simulink model "OORT"  (Simulink 7.6)
settings: Solver=ode3  SolverMode=SingleTasking  StartTime=0.0  StopTime=1.2  FixedStep=2e-5  RelTol=1e-4  AbsTol=1e-6
undefined symbols (not defined in the file or in its folder): DAB, den, elements, num
libraries: powerlib x179, powerlib_extras x6
(part 3 of 4)

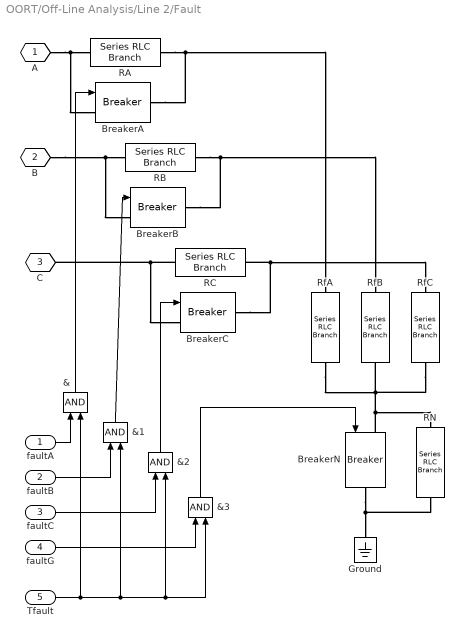
== system OORT/Off-Line Analysis/Line 2/Fault ==
  faultA : Inport
  faultB : Inport  Port=2
  faultC : Inport  Port=3
  faultG : Inport  Port=4
  Tfault : Inport  Port=5
  &{,1..3} (4 alike) : Logic
  BreakerA : powerlib/Elements/Breaker  DialogController=POWERSYS.PowerSysDialog  SystemSampleTime=-1  BreakerResistance=0.01  InitialState=0  SnubberResistance=1e6  SnubberCapacitance=inf  SwitchingTimes="[ 1/60  5/60 ]"  External=on  Measurements=None  MoreParameters=off  NoBreakLoop=off
  BreakerB : powerlib/Elements/Breaker  DialogController=POWERSYS.PowerSysDialog  SystemSampleTime=-1  BreakerResistance=0.01  InitialState=0  SnubberResistance=1e6  SnubberCapacitance=inf  SwitchingTimes="[ 1/60  5/60 ]"  External=on  Measurements=None  MoreParameters=off  NoBreakLoop=off
  BreakerC : powerlib/Elements/Breaker  DialogController=POWERSYS.PowerSysDialog  SystemSampleTime=-1  BreakerResistance=0.01  InitialState=0  SnubberResistance=1e6  SnubberCapacitance=inf  SwitchingTimes="[ 1/60  5/60 ]"  External=on  Measurements=None  MoreParameters=off  NoBreakLoop=off
  BreakerN : powerlib/Elements/Breaker  DialogController=POWERSYS.PowerSysDialog  SystemSampleTime=-1  BreakerResistance=0.01  InitialState=0  SnubberResistance=1e6  SnubberCapacitance=inf  SwitchingTimes="[ 1/60  5/60 ]"  External=on  Measurements=None  MoreParameters=off  NoBreakLoop=off
  Ground : powerlib/Elements/Ground  DialogController=POWERSYS.PowerSysDialog  PhysicalDomain=powersysdomain  SubClassName=unknown  LeftPortType=p1  RightPortType=p1  LConnTagsString=a
  RA : powerlib/Elements/Series RLC Branch  DialogController=POWERSYS.PowerSysDialog  PhysicalDomain=powersysdomain  SubClassName=unknown  LeftPortType=p1  RightPortType=p1  LConnTagsString=__new0  RConnTagsString=__new0  BranchType=R  Resistance=10000  Inductance=1e-3  SetiL0=off  InitialCurrent=0  Capacitance=1e-6  Setx0=off  InitialVoltage=0  Measurements=None
  RB : powerlib/Elements/Series RLC Branch  DialogController=POWERSYS.PowerSysDialog  PhysicalDomain=powersysdomain  SubClassName=unknown  LeftPortType=p1  RightPortType=p1  LConnTagsString=__new0  RConnTagsString=__new0  BranchType=R  Resistance=10000  Inductance=1e-3  SetiL0=off  InitialCurrent=0  Capacitance=1e-6  Setx0=off  InitialVoltage=0  Measurements=None
  RC : powerlib/Elements/Series RLC Branch  DialogController=POWERSYS.PowerSysDialog  PhysicalDomain=powersysdomain  SubClassName=unknown  LeftPortType=p1  RightPortType=p1  LConnTagsString=__new0  RConnTagsString=__new0  BranchType=R  Resistance=10000  Inductance=1e-3  SetiL0=off  InitialCurrent=0  Capacitance=1e-6  Setx0=off  InitialVoltage=0  Measurements=None
  RN : powerlib/Elements/Series RLC Branch  DialogController=POWERSYS.PowerSysDialog  PhysicalDomain=powersysdomain  SubClassName=unknown  LeftPortType=p1  RightPortType=p1  LConnTagsString=__new0  RConnTagsString=__new0  BranchType=R  Resistance=10000  Inductance=1e-3  SetiL0=off  InitialCurrent=0  Capacitance=1e-6  Setx0=off  InitialVoltage=0  Measurements=None
  RfA : powerlib/Elements/Series RLC Branch  DialogController=POWERSYS.PowerSysDialog  PhysicalDomain=powersysdomain  SubClassName=unknown  LeftPortType=p1  RightPortType=p1  LConnTagsString=__new0  RConnTagsString=__new0  BranchType=R  Resistance=faultR  Inductance=1e-3  SetiL0=off  InitialCurrent=0  Capacitance=1e-6  Setx0=off  InitialVoltage=0  Measurements=None
  RfB : powerlib/Elements/Series RLC Branch  DialogController=POWERSYS.PowerSysDialog  PhysicalDomain=powersysdomain  SubClassName=unknown  LeftPortType=p1  RightPortType=p1  LConnTagsString=__new0  RConnTagsString=__new0  BranchType=R  Resistance=faultR  Inductance=1e-3  SetiL0=off  InitialCurrent=0  Capacitance=1e-6  Setx0=off  InitialVoltage=0  Measurements=None
  RfC : powerlib/Elements/Series RLC Branch  DialogController=POWERSYS.PowerSysDialog  PhysicalDomain=powersysdomain  SubClassName=unknown  LeftPortType=p1  RightPortType=p1  LConnTagsString=__new0  RConnTagsString=__new0  BranchType=R  Resistance=faultR  Inductance=1e-3  SetiL0=off  InitialCurrent=0  Capacitance=1e-6  Setx0=off  InitialVoltage=0  Measurements=None
  A : PMIOPort  Tag=PMCPort  Port=1  Side=Left
  B : PMIOPort  Tag=PMCPort  Port=2  Side=Left
  C : PMIOPort  Tag=PMCPort  Port=3  Side=Left
  wires:
  faultA/1 -> &/1
  faultB/1 -> &1/1
  faultC/1 -> &2/1
  faultG/1 -> &3/1
  Tfault/1 -> &3/2, &2/2, &1/2, &/2
  &3/1 -> BreakerN/1
  &/1 -> BreakerA/1
  &1/1 -> BreakerB/1
  &2/1 -> BreakerC/1
  connections:
  B/RConn1 -- RB/LConn1 -- BreakerB/LConn1
  A/RConn1 -- BreakerA/LConn1 -- RA/LConn1
  RC/LConn1 -- C/RConn1 -- BreakerC/LConn1
  BreakerC/RConn1 -- RC/RConn1 -- RfC/LConn1
  RB/RConn1 -- RfB/LConn1 -- BreakerB/RConn1
  RA/RConn1 -- RfA/LConn1 -- BreakerA/RConn1
  BreakerN/LConn1 -- RN/LConn1 -- RfB/RConn1 -- RfA/RConn1 -- RfC/RConn1
  BreakerN/RConn1 -- Ground/LConn1 -- RN/RConn1

== system OORT/Off-Line Analysis/Line 2/Fault Selector ==
  "  " : Constant  Value=faultType
  "  +" : Logic  Operator=OR  Inputs=7
  " +" : Logic  Operator=OR  Inputs=5
  + : Logic  Operator=OR  Inputs=5
  "+ " : Logic  Operator=OR  Inputs=6
  A-B-C : Fcn  Expr=(u(1)==8)
  A-B-C-G : Fcn  Expr=(u(1)==9)
  A-G : Fcn  Expr=(u(1)==1)
  B-C : Fcn  Expr=(u(1)==4)
  B-C-G : Fcn  Expr=(u(1)==5)
  B-G : Fcn  Expr=(u(1)==2)
  C-A : Fcn  Expr=(u(1)==6)
  C-A-G : Fcn  Expr=(u(1)==7)
  C-G : Fcn  Expr=(u(1)==3)
  faultA : Outport  InitialOutput=0
  faultB : Outport  Port=2  InitialOutput=0
  faultC : Outport  Port=3  InitialOutput=0
  faultG : Outport  Port=4  InitialOutput=0
  wires:
  "  "/1 -> C-G/1, A-G/1, B-G/1, B-C/1, C-A/1, C-A-G/1, A-B-C/1, A-B-C-G/1, B-C-G/1
  +/1 -> faultA/1
  " +"/1 -> faultB/1
  "  +"/1 -> faultC/1
  "+ "/1 -> faultG/1
  A-G/1 -> "+ "/1, +/1
  C-A/1 -> "  +"/4, +/2
  B-G/1 -> " +"/1, "+ "/2
  B-C/1 -> "  +"/2, " +"/2
  B-C-G/1 -> "  +"/3, "+ "/4, " +"/3
  C-G/1 -> "  +"/1, "+ "/3
  C-A-G/1 -> "  +"/5, "+ "/5, +/3
  A-B-C-G/1 -> " +"/5, "  +"/7, "+ "/6, +/5
  A-B-C/1 -> " +"/4, "  +"/6, +/4

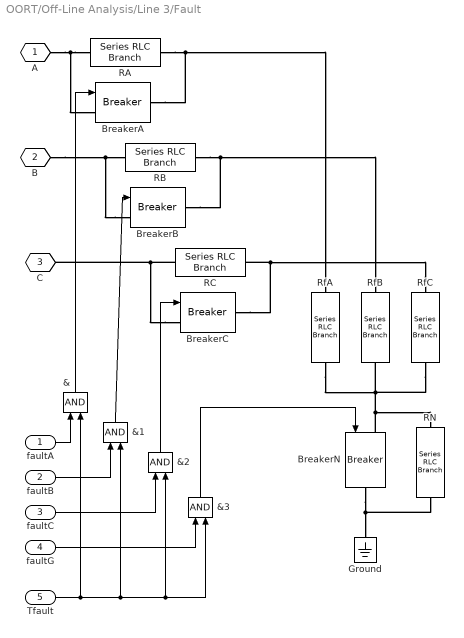
== system OORT/Off-Line Analysis/Line 3/Fault ==
  faultA : Inport
  faultB : Inport  Port=2
  faultC : Inport  Port=3
  faultG : Inport  Port=4
  Tfault : Inport  Port=5
  &{,1..3} (4 alike) : Logic
  BreakerA : powerlib/Elements/Breaker  DialogController=POWERSYS.PowerSysDialog  SystemSampleTime=-1  BreakerResistance=0.01  InitialState=0  SnubberResistance=1e6  SnubberCapacitance=inf  SwitchingTimes="[ 1/60  5/60 ]"  External=on  Measurements=None  MoreParameters=off  NoBreakLoop=off
  BreakerB : powerlib/Elements/Breaker  DialogController=POWERSYS.PowerSysDialog  SystemSampleTime=-1  BreakerResistance=0.01  InitialState=0  SnubberResistance=1e6  SnubberCapacitance=inf  SwitchingTimes="[ 1/60  5/60 ]"  External=on  Measurements=None  MoreParameters=off  NoBreakLoop=off
  BreakerC : powerlib/Elements/Breaker  DialogController=POWERSYS.PowerSysDialog  SystemSampleTime=-1  BreakerResistance=0.01  InitialState=0  SnubberResistance=1e6  SnubberCapacitance=inf  SwitchingTimes="[ 1/60  5/60 ]"  External=on  Measurements=None  MoreParameters=off  NoBreakLoop=off
  BreakerN : powerlib/Elements/Breaker  DialogController=POWERSYS.PowerSysDialog  SystemSampleTime=-1  BreakerResistance=0.01  InitialState=0  SnubberResistance=1e6  SnubberCapacitance=inf  SwitchingTimes="[ 1/60  5/60 ]"  External=on  Measurements=None  MoreParameters=off  NoBreakLoop=off
  Ground : powerlib/Elements/Ground  DialogController=POWERSYS.PowerSysDialog  PhysicalDomain=powersysdomain  SubClassName=unknown  LeftPortType=p1  RightPortType=p1  LConnTagsString=a
  RA : powerlib/Elements/Series RLC Branch  DialogController=POWERSYS.PowerSysDialog  PhysicalDomain=powersysdomain  SubClassName=unknown  LeftPortType=p1  RightPortType=p1  LConnTagsString=__new0  RConnTagsString=__new0  BranchType=R  Resistance=10000  Inductance=1e-3  SetiL0=off  InitialCurrent=0  Capacitance=1e-6  Setx0=off  InitialVoltage=0  Measurements=None
  RB : powerlib/Elements/Series RLC Branch  DialogController=POWERSYS.PowerSysDialog  PhysicalDomain=powersysdomain  SubClassName=unknown  LeftPortType=p1  RightPortType=p1  LConnTagsString=__new0  RConnTagsString=__new0  BranchType=R  Resistance=10000  Inductance=1e-3  SetiL0=off  InitialCurrent=0  Capacitance=1e-6  Setx0=off  InitialVoltage=0  Measurements=None
  RC : powerlib/Elements/Series RLC Branch  DialogController=POWERSYS.PowerSysDialog  PhysicalDomain=powersysdomain  SubClassName=unknown  LeftPortType=p1  RightPortType=p1  LConnTagsString=__new0  RConnTagsString=__new0  BranchType=R  Resistance=10000  Inductance=1e-3  SetiL0=off  InitialCurrent=0  Capacitance=1e-6  Setx0=off  InitialVoltage=0  Measurements=None
  RN : powerlib/Elements/Series RLC Branch  DialogController=POWERSYS.PowerSysDialog  PhysicalDomain=powersysdomain  SubClassName=unknown  LeftPortType=p1  RightPortType=p1  LConnTagsString=__new0  RConnTagsString=__new0  BranchType=R  Resistance=10000  Inductance=1e-3  SetiL0=off  InitialCurrent=0  Capacitance=1e-6  Setx0=off  InitialVoltage=0  Measurements=None
  RfA : powerlib/Elements/Series RLC Branch  DialogController=POWERSYS.PowerSysDialog  PhysicalDomain=powersysdomain  SubClassName=unknown  LeftPortType=p1  RightPortType=p1  LConnTagsString=__new0  RConnTagsString=__new0  BranchType=R  Resistance=faultR  Inductance=1e-3  SetiL0=off  InitialCurrent=0  Capacitance=1e-6  Setx0=off  InitialVoltage=0  Measurements=None
  RfB : powerlib/Elements/Series RLC Branch  DialogController=POWERSYS.PowerSysDialog  PhysicalDomain=powersysdomain  SubClassName=unknown  LeftPortType=p1  RightPortType=p1  LConnTagsString=__new0  RConnTagsString=__new0  BranchType=R  Resistance=faultR  Inductance=1e-3  SetiL0=off  InitialCurrent=0  Capacitance=1e-6  Setx0=off  InitialVoltage=0  Measurements=None
  RfC : powerlib/Elements/Series RLC Branch  DialogController=POWERSYS.PowerSysDialog  PhysicalDomain=powersysdomain  SubClassName=unknown  LeftPortType=p1  RightPortType=p1  LConnTagsString=__new0  RConnTagsString=__new0  BranchType=R  Resistance=faultR  Inductance=1e-3  SetiL0=off  InitialCurrent=0  Capacitance=1e-6  Setx0=off  InitialVoltage=0  Measurements=None
  A : PMIOPort  Tag=PMCPort  Port=1  Side=Left
  B : PMIOPort  Tag=PMCPort  Port=2  Side=Left
  C : PMIOPort  Tag=PMCPort  Port=3  Side=Left
  wires:
  &2/1 -> BreakerC/1
  &1/1 -> BreakerB/1
  &/1 -> BreakerA/1
  &3/1 -> BreakerN/1
  Tfault/1 -> &/2, &1/2, &2/2, &3/2
  faultG/1 -> &3/1
  faultC/1 -> &2/1
  faultB/1 -> &1/1
  faultA/1 -> &/1
  connections:
  RN/RConn1 -- Ground/LConn1 -- BreakerN/RConn1
  RfC/RConn1 -- RfA/RConn1 -- RfB/RConn1 -- RN/LConn1 -- BreakerN/LConn1
  BreakerA/RConn1 -- RfA/LConn1 -- RA/RConn1
  BreakerB/RConn1 -- RfB/LConn1 -- RB/RConn1
  RfC/LConn1 -- RC/RConn1 -- BreakerC/RConn1
  BreakerC/LConn1 -- C/RConn1 -- RC/LConn1
  RA/LConn1 -- BreakerA/LConn1 -- A/RConn1
  BreakerB/LConn1 -- RB/LConn1 -- B/RConn1

== system OORT/Off-Line Analysis/Line 3/Fault Selector ==
  "  " : Constant  Value=faultType
  "  +" : Logic  Operator=OR  Inputs=7
  " +" : Logic  Operator=OR  Inputs=5
  + : Logic  Operator=OR  Inputs=5
  "+ " : Logic  Operator=OR  Inputs=6
  A-B-C : Fcn  Expr=(u(1)==8)
  A-B-C-G : Fcn  Expr=(u(1)==9)
  A-G : Fcn  Expr=(u(1)==1)
  B-C : Fcn  Expr=(u(1)==4)
  B-C-G : Fcn  Expr=(u(1)==5)
  B-G : Fcn  Expr=(u(1)==2)
  C-A : Fcn  Expr=(u(1)==6)
  C-A-G : Fcn  Expr=(u(1)==7)
  C-G : Fcn  Expr=(u(1)==3)
  faultA : Outport  InitialOutput=0
  faultB : Outport  Port=2  InitialOutput=0
  faultC : Outport  Port=3  InitialOutput=0
  faultG : Outport  Port=4  InitialOutput=0
  wires:
  A-B-C/1 -> +/4, "  +"/6, " +"/4
  A-B-C-G/1 -> +/5, "+ "/6, "  +"/7, " +"/5
  C-A-G/1 -> +/3, "+ "/5, "  +"/5
  C-G/1 -> "+ "/3, "  +"/1
  B-C-G/1 -> " +"/3, "+ "/4, "  +"/3
  B-C/1 -> " +"/2, "  +"/2
  B-G/1 -> "+ "/2, " +"/1
  C-A/1 -> +/2, "  +"/4
  A-G/1 -> +/1, "+ "/1
  "+ "/1 -> faultG/1
  "  +"/1 -> faultC/1
  " +"/1 -> faultB/1
  +/1 -> faultA/1
  "  "/1 -> B-C-G/1, A-B-C-G/1, A-B-C/1, C-A-G/1, C-A/1, B-C/1, B-G/1, A-G/1, C-G/1

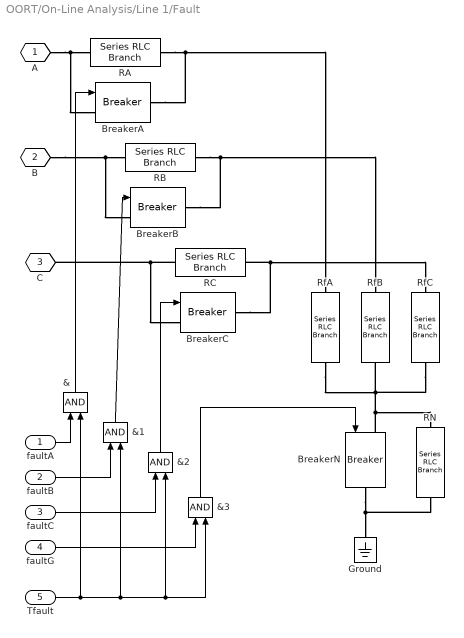
== system OORT/On-Line Analysis/Line 1/Fault ==
  faultA : Inport
  faultB : Inport  Port=2
  faultC : Inport  Port=3
  faultG : Inport  Port=4
  Tfault : Inport  Port=5
  &{,1..3} (4 alike) : Logic
  BreakerA : powerlib/Elements/Breaker  DialogController=POWERSYS.PowerSysDialog  SystemSampleTime=-1  BreakerResistance=0.01  InitialState=0  SnubberResistance=1e6  SnubberCapacitance=inf  SwitchingTimes="[ 1/60  5/60 ]"  External=on  Measurements=None  MoreParameters=off  NoBreakLoop=off
  BreakerB : powerlib/Elements/Breaker  DialogController=POWERSYS.PowerSysDialog  SystemSampleTime=-1  BreakerResistance=0.01  InitialState=0  SnubberResistance=1e6  SnubberCapacitance=inf  SwitchingTimes="[ 1/60  5/60 ]"  External=on  Measurements=None  MoreParameters=off  NoBreakLoop=off
  BreakerC : powerlib/Elements/Breaker  DialogController=POWERSYS.PowerSysDialog  SystemSampleTime=-1  BreakerResistance=0.01  InitialState=0  SnubberResistance=1e6  SnubberCapacitance=inf  SwitchingTimes="[ 1/60  5/60 ]"  External=on  Measurements=None  MoreParameters=off  NoBreakLoop=off
  BreakerN : powerlib/Elements/Breaker  DialogController=POWERSYS.PowerSysDialog  SystemSampleTime=-1  BreakerResistance=0.01  InitialState=0  SnubberResistance=1e6  SnubberCapacitance=inf  SwitchingTimes="[ 1/60  5/60 ]"  External=on  Measurements=None  MoreParameters=off  NoBreakLoop=off
  Ground : powerlib/Elements/Ground  DialogController=POWERSYS.PowerSysDialog  PhysicalDomain=powersysdomain  SubClassName=unknown  LeftPortType=p1  RightPortType=p1  LConnTagsString=a
  RA : powerlib/Elements/Series RLC Branch  DialogController=POWERSYS.PowerSysDialog  PhysicalDomain=powersysdomain  SubClassName=unknown  LeftPortType=p1  RightPortType=p1  LConnTagsString=__new0  RConnTagsString=__new0  BranchType=R  Resistance=10000  Inductance=1e-3  SetiL0=off  InitialCurrent=0  Capacitance=1e-6  Setx0=off  InitialVoltage=0  Measurements=None
  RB : powerlib/Elements/Series RLC Branch  DialogController=POWERSYS.PowerSysDialog  PhysicalDomain=powersysdomain  SubClassName=unknown  LeftPortType=p1  RightPortType=p1  LConnTagsString=__new0  RConnTagsString=__new0  BranchType=R  Resistance=10000  Inductance=1e-3  SetiL0=off  InitialCurrent=0  Capacitance=1e-6  Setx0=off  InitialVoltage=0  Measurements=None
  RC : powerlib/Elements/Series RLC Branch  DialogController=POWERSYS.PowerSysDialog  PhysicalDomain=powersysdomain  SubClassName=unknown  LeftPortType=p1  RightPortType=p1  LConnTagsString=__new0  RConnTagsString=__new0  BranchType=R  Resistance=10000  Inductance=1e-3  SetiL0=off  InitialCurrent=0  Capacitance=1e-6  Setx0=off  InitialVoltage=0  Measurements=None
  RN : powerlib/Elements/Series RLC Branch  DialogController=POWERSYS.PowerSysDialog  PhysicalDomain=powersysdomain  SubClassName=unknown  LeftPortType=p1  RightPortType=p1  LConnTagsString=__new0  RConnTagsString=__new0  BranchType=R  Resistance=10000  Inductance=1e-3  SetiL0=off  InitialCurrent=0  Capacitance=1e-6  Setx0=off  InitialVoltage=0  Measurements=None
  RfA : powerlib/Elements/Series RLC Branch  DialogController=POWERSYS.PowerSysDialog  PhysicalDomain=powersysdomain  SubClassName=unknown  LeftPortType=p1  RightPortType=p1  LConnTagsString=__new0  RConnTagsString=__new0  BranchType=R  Resistance=faultR  Inductance=1e-3  SetiL0=off  InitialCurrent=0  Capacitance=1e-6  Setx0=off  InitialVoltage=0  Measurements=None
  RfB : powerlib/Elements/Series RLC Branch  DialogController=POWERSYS.PowerSysDialog  PhysicalDomain=powersysdomain  SubClassName=unknown  LeftPortType=p1  RightPortType=p1  LConnTagsString=__new0  RConnTagsString=__new0  BranchType=R  Resistance=faultR  Inductance=1e-3  SetiL0=off  InitialCurrent=0  Capacitance=1e-6  Setx0=off  InitialVoltage=0  Measurements=None
  RfC : powerlib/Elements/Series RLC Branch  DialogController=POWERSYS.PowerSysDialog  PhysicalDomain=powersysdomain  SubClassName=unknown  LeftPortType=p1  RightPortType=p1  LConnTagsString=__new0  RConnTagsString=__new0  BranchType=R  Resistance=faultR  Inductance=1e-3  SetiL0=off  InitialCurrent=0  Capacitance=1e-6  Setx0=off  InitialVoltage=0  Measurements=None
  A : PMIOPort  Tag=PMCPort  Port=1  Side=Left
  B : PMIOPort  Tag=PMCPort  Port=2  Side=Left
  C : PMIOPort  Tag=PMCPort  Port=3  Side=Left
  wires:
  faultA/1 -> &/1
  faultB/1 -> &1/1
  faultC/1 -> &2/1
  faultG/1 -> &3/1
  Tfault/1 -> &3/2, &2/2, &1/2, &/2
  &3/1 -> BreakerN/1
  &/1 -> BreakerA/1
  &1/1 -> BreakerB/1
  &2/1 -> BreakerC/1
  connections:
  B/RConn1 -- RB/LConn1 -- BreakerB/LConn1
  A/RConn1 -- BreakerA/LConn1 -- RA/LConn1
  RC/LConn1 -- C/RConn1 -- BreakerC/LConn1
  BreakerC/RConn1 -- RC/RConn1 -- RfC/LConn1
  RB/RConn1 -- RfB/LConn1 -- BreakerB/RConn1
  RA/RConn1 -- RfA/LConn1 -- BreakerA/RConn1
  BreakerN/LConn1 -- RN/LConn1 -- RfB/RConn1 -- RfA/RConn1 -- RfC/RConn1
  BreakerN/RConn1 -- Ground/LConn1 -- RN/RConn1

== system OORT/On-Line Analysis/Line 1/Fault Selector ==
  "  " : Constant  Value=faultType
  "  +" : Logic  Operator=OR  Inputs=7
  " +" : Logic  Operator=OR  Inputs=5
  + : Logic  Operator=OR  Inputs=5
  "+ " : Logic  Operator=OR  Inputs=6
  A-B-C : Fcn  Expr=(u(1)==8)
  A-B-C-G : Fcn  Expr=(u(1)==9)
  A-G : Fcn  Expr=(u(1)==1)
  B-C : Fcn  Expr=(u(1)==4)
  B-C-G : Fcn  Expr=(u(1)==5)
  B-G : Fcn  Expr=(u(1)==2)
  C-A : Fcn  Expr=(u(1)==6)
  C-A-G : Fcn  Expr=(u(1)==7)
  C-G : Fcn  Expr=(u(1)==3)
  faultA : Outport  InitialOutput=0
  faultB : Outport  Port=2  InitialOutput=0
  faultC : Outport  Port=3  InitialOutput=0
  faultG : Outport  Port=4  InitialOutput=0
  wires:
  "  "/1 -> C-G/1, A-G/1, B-G/1, B-C/1, C-A/1, C-A-G/1, A-B-C/1, A-B-C-G/1, B-C-G/1
  +/1 -> faultA/1
  " +"/1 -> faultB/1
  "  +"/1 -> faultC/1
  "+ "/1 -> faultG/1
  A-G/1 -> "+ "/1, +/1
  C-A/1 -> "  +"/4, +/2
  B-G/1 -> " +"/1, "+ "/2
  B-C/1 -> "  +"/2, " +"/2
  B-C-G/1 -> "  +"/3, "+ "/4, " +"/3
  C-G/1 -> "  +"/1, "+ "/3
  C-A-G/1 -> "  +"/5, "+ "/5, +/3
  A-B-C-G/1 -> " +"/5, "  +"/7, "+ "/6, +/5
  A-B-C/1 -> " +"/4, "  +"/6, +/4

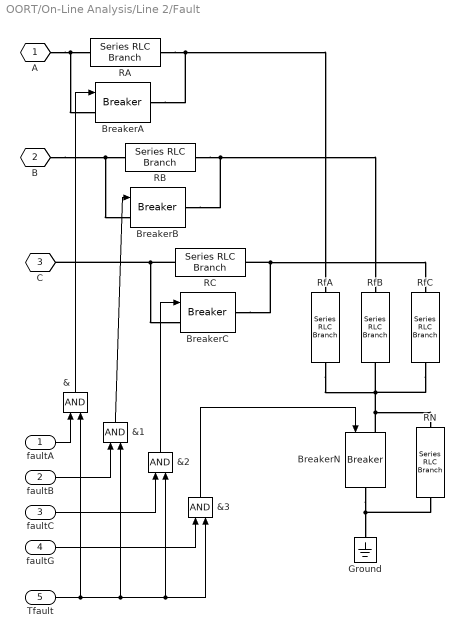
== system OORT/On-Line Analysis/Line 2/Fault ==
  faultA : Inport
  faultB : Inport  Port=2
  faultC : Inport  Port=3
  faultG : Inport  Port=4
  Tfault : Inport  Port=5
  &{,1..3} (4 alike) : Logic
  BreakerA : powerlib/Elements/Breaker  DialogController=POWERSYS.PowerSysDialog  SystemSampleTime=-1  BreakerResistance=0.01  InitialState=0  SnubberResistance=1e6  SnubberCapacitance=inf  SwitchingTimes="[ 1/60  5/60 ]"  External=on  Measurements=None  MoreParameters=off  NoBreakLoop=off
  BreakerB : powerlib/Elements/Breaker  DialogController=POWERSYS.PowerSysDialog  SystemSampleTime=-1  BreakerResistance=0.01  InitialState=0  SnubberResistance=1e6  SnubberCapacitance=inf  SwitchingTimes="[ 1/60  5/60 ]"  External=on  Measurements=None  MoreParameters=off  NoBreakLoop=off
  BreakerC : powerlib/Elements/Breaker  DialogController=POWERSYS.PowerSysDialog  SystemSampleTime=-1  BreakerResistance=0.01  InitialState=0  SnubberResistance=1e6  SnubberCapacitance=inf  SwitchingTimes="[ 1/60  5/60 ]"  External=on  Measurements=None  MoreParameters=off  NoBreakLoop=off
  BreakerN : powerlib/Elements/Breaker  DialogController=POWERSYS.PowerSysDialog  SystemSampleTime=-1  BreakerResistance=0.01  InitialState=0  SnubberResistance=1e6  SnubberCapacitance=inf  SwitchingTimes="[ 1/60  5/60 ]"  External=on  Measurements=None  MoreParameters=off  NoBreakLoop=off
  Ground : powerlib/Elements/Ground  DialogController=POWERSYS.PowerSysDialog  PhysicalDomain=powersysdomain  SubClassName=unknown  LeftPortType=p1  RightPortType=p1  LConnTagsString=a
  RA : powerlib/Elements/Series RLC Branch  DialogController=POWERSYS.PowerSysDialog  PhysicalDomain=powersysdomain  SubClassName=unknown  LeftPortType=p1  RightPortType=p1  LConnTagsString=__new0  RConnTagsString=__new0  BranchType=R  Resistance=10000  Inductance=1e-3  SetiL0=off  InitialCurrent=0  Capacitance=1e-6  Setx0=off  InitialVoltage=0  Measurements=None
  RB : powerlib/Elements/Series RLC Branch  DialogController=POWERSYS.PowerSysDialog  PhysicalDomain=powersysdomain  SubClassName=unknown  LeftPortType=p1  RightPortType=p1  LConnTagsString=__new0  RConnTagsString=__new0  BranchType=R  Resistance=10000  Inductance=1e-3  SetiL0=off  InitialCurrent=0  Capacitance=1e-6  Setx0=off  InitialVoltage=0  Measurements=None
  RC : powerlib/Elements/Series RLC Branch  DialogController=POWERSYS.PowerSysDialog  PhysicalDomain=powersysdomain  SubClassName=unknown  LeftPortType=p1  RightPortType=p1  LConnTagsString=__new0  RConnTagsString=__new0  BranchType=R  Resistance=10000  Inductance=1e-3  SetiL0=off  InitialCurrent=0  Capacitance=1e-6  Setx0=off  InitialVoltage=0  Measurements=None
  RN : powerlib/Elements/Series RLC Branch  DialogController=POWERSYS.PowerSysDialog  PhysicalDomain=powersysdomain  SubClassName=unknown  LeftPortType=p1  RightPortType=p1  LConnTagsString=__new0  RConnTagsString=__new0  BranchType=R  Resistance=10000  Inductance=1e-3  SetiL0=off  InitialCurrent=0  Capacitance=1e-6  Setx0=off  InitialVoltage=0  Measurements=None
  RfA : powerlib/Elements/Series RLC Branch  DialogController=POWERSYS.PowerSysDialog  PhysicalDomain=powersysdomain  SubClassName=unknown  LeftPortType=p1  RightPortType=p1  LConnTagsString=__new0  RConnTagsString=__new0  BranchType=R  Resistance=faultR  Inductance=1e-3  SetiL0=off  InitialCurrent=0  Capacitance=1e-6  Setx0=off  InitialVoltage=0  Measurements=None
  RfB : powerlib/Elements/Series RLC Branch  DialogController=POWERSYS.PowerSysDialog  PhysicalDomain=powersysdomain  SubClassName=unknown  LeftPortType=p1  RightPortType=p1  LConnTagsString=__new0  RConnTagsString=__new0  BranchType=R  Resistance=faultR  Inductance=1e-3  SetiL0=off  InitialCurrent=0  Capacitance=1e-6  Setx0=off  InitialVoltage=0  Measurements=None
  RfC : powerlib/Elements/Series RLC Branch  DialogController=POWERSYS.PowerSysDialog  PhysicalDomain=powersysdomain  SubClassName=unknown  LeftPortType=p1  RightPortType=p1  LConnTagsString=__new0  RConnTagsString=__new0  BranchType=R  Resistance=faultR  Inductance=1e-3  SetiL0=off  InitialCurrent=0  Capacitance=1e-6  Setx0=off  InitialVoltage=0  Measurements=None
  A : PMIOPort  Tag=PMCPort  Port=1  Side=Left
  B : PMIOPort  Tag=PMCPort  Port=2  Side=Left
  C : PMIOPort  Tag=PMCPort  Port=3  Side=Left
  wires:
  faultA/1 -> &/1
  faultB/1 -> &1/1
  faultC/1 -> &2/1
  faultG/1 -> &3/1
  Tfault/1 -> &3/2, &2/2, &1/2, &/2
  &3/1 -> BreakerN/1
  &/1 -> BreakerA/1
  &1/1 -> BreakerB/1
  &2/1 -> BreakerC/1
  connections:
  B/RConn1 -- RB/LConn1 -- BreakerB/LConn1
  A/RConn1 -- BreakerA/LConn1 -- RA/LConn1
  RC/LConn1 -- C/RConn1 -- BreakerC/LConn1
  BreakerC/RConn1 -- RC/RConn1 -- RfC/LConn1
  RB/RConn1 -- RfB/LConn1 -- BreakerB/RConn1
  RA/RConn1 -- RfA/LConn1 -- BreakerA/RConn1
  BreakerN/LConn1 -- RN/LConn1 -- RfB/RConn1 -- RfA/RConn1 -- RfC/RConn1
  BreakerN/RConn1 -- Ground/LConn1 -- RN/RConn1

== system OORT/On-Line Analysis/Line 2/Fault Selector ==
  "  " : Constant  Value=faultType
  "  +" : Logic  Operator=OR  Inputs=7
  " +" : Logic  Operator=OR  Inputs=5
  + : Logic  Operator=OR  Inputs=5
  "+ " : Logic  Operator=OR  Inputs=6
  A-B-C : Fcn  Expr=(u(1)==8)
  A-B-C-G : Fcn  Expr=(u(1)==9)
  A-G : Fcn  Expr=(u(1)==1)
  B-C : Fcn  Expr=(u(1)==4)
  B-C-G : Fcn  Expr=(u(1)==5)
  B-G : Fcn  Expr=(u(1)==2)
  C-A : Fcn  Expr=(u(1)==6)
  C-A-G : Fcn  Expr=(u(1)==7)
  C-G : Fcn  Expr=(u(1)==3)
  faultA : Outport  InitialOutput=0
  faultB : Outport  Port=2  InitialOutput=0
  faultC : Outport  Port=3  InitialOutput=0
  faultG : Outport  Port=4  InitialOutput=0
  wires:
  "  "/1 -> C-G/1, A-G/1, B-G/1, B-C/1, C-A/1, C-A-G/1, A-B-C/1, A-B-C-G/1, B-C-G/1
  +/1 -> faultA/1
  " +"/1 -> faultB/1
  "  +"/1 -> faultC/1
  "+ "/1 -> faultG/1
  A-G/1 -> "+ "/1, +/1
  C-A/1 -> "  +"/4, +/2
  B-G/1 -> " +"/1, "+ "/2
  B-C/1 -> "  +"/2, " +"/2
  B-C-G/1 -> "  +"/3, "+ "/4, " +"/3
  C-G/1 -> "  +"/1, "+ "/3
  C-A-G/1 -> "  +"/5, "+ "/5, +/3
  A-B-C-G/1 -> " +"/5, "  +"/7, "+ "/6, +/5
  A-B-C/1 -> " +"/4, "  +"/6, +/4

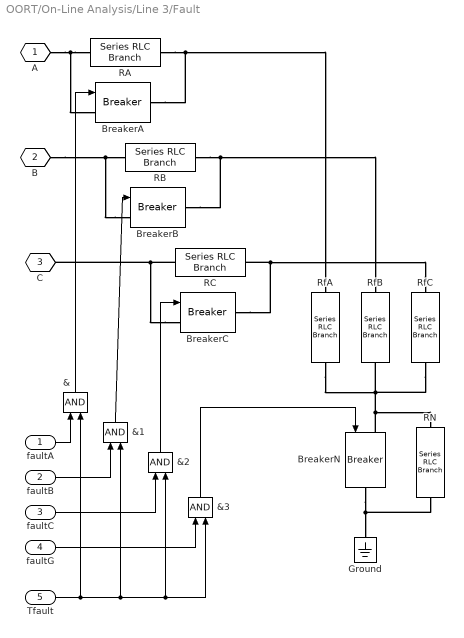
== system OORT/On-Line Analysis/Line 3/Fault ==
  faultA : Inport
  faultB : Inport  Port=2
  faultC : Inport  Port=3
  faultG : Inport  Port=4
  Tfault : Inport  Port=5
  &{,1..3} (4 alike) : Logic
  BreakerA : powerlib/Elements/Breaker  DialogController=POWERSYS.PowerSysDialog  SystemSampleTime=-1  BreakerResistance=0.01  InitialState=0  SnubberResistance=1e6  SnubberCapacitance=inf  SwitchingTimes="[ 1/60  5/60 ]"  External=on  Measurements=None  MoreParameters=off  NoBreakLoop=off
  BreakerB : powerlib/Elements/Breaker  DialogController=POWERSYS.PowerSysDialog  SystemSampleTime=-1  BreakerResistance=0.01  InitialState=0  SnubberResistance=1e6  SnubberCapacitance=inf  SwitchingTimes="[ 1/60  5/60 ]"  External=on  Measurements=None  MoreParameters=off  NoBreakLoop=off
  BreakerC : powerlib/Elements/Breaker  DialogController=POWERSYS.PowerSysDialog  SystemSampleTime=-1  BreakerResistance=0.01  InitialState=0  SnubberResistance=1e6  SnubberCapacitance=inf  SwitchingTimes="[ 1/60  5/60 ]"  External=on  Measurements=None  MoreParameters=off  NoBreakLoop=off
  BreakerN : powerlib/Elements/Breaker  DialogController=POWERSYS.PowerSysDialog  SystemSampleTime=-1  BreakerResistance=0.01  InitialState=0  SnubberResistance=1e6  SnubberCapacitance=inf  SwitchingTimes="[ 1/60  5/60 ]"  External=on  Measurements=None  MoreParameters=off  NoBreakLoop=off
  Ground : powerlib/Elements/Ground  DialogController=POWERSYS.PowerSysDialog  PhysicalDomain=powersysdomain  SubClassName=unknown  LeftPortType=p1  RightPortType=p1  LConnTagsString=a
  RA : powerlib/Elements/Series RLC Branch  DialogController=POWERSYS.PowerSysDialog  PhysicalDomain=powersysdomain  SubClassName=unknown  LeftPortType=p1  RightPortType=p1  LConnTagsString=__new0  RConnTagsString=__new0  BranchType=R  Resistance=10000  Inductance=1e-3  SetiL0=off  InitialCurrent=0  Capacitance=1e-6  Setx0=off  InitialVoltage=0  Measurements=None
  RB : powerlib/Elements/Series RLC Branch  DialogController=POWERSYS.PowerSysDialog  PhysicalDomain=powersysdomain  SubClassName=unknown  LeftPortType=p1  RightPortType=p1  LConnTagsString=__new0  RConnTagsString=__new0  BranchType=R  Resistance=10000  Inductance=1e-3  SetiL0=off  InitialCurrent=0  Capacitance=1e-6  Setx0=off  InitialVoltage=0  Measurements=None
  RC : powerlib/Elements/Series RLC Branch  DialogController=POWERSYS.PowerSysDialog  PhysicalDomain=powersysdomain  SubClassName=unknown  LeftPortType=p1  RightPortType=p1  LConnTagsString=__new0  RConnTagsString=__new0  BranchType=R  Resistance=10000  Inductance=1e-3  SetiL0=off  InitialCurrent=0  Capacitance=1e-6  Setx0=off  InitialVoltage=0  Measurements=None
  RN : powerlib/Elements/Series RLC Branch  DialogController=POWERSYS.PowerSysDialog  PhysicalDomain=powersysdomain  SubClassName=unknown  LeftPortType=p1  RightPortType=p1  LConnTagsString=__new0  RConnTagsString=__new0  BranchType=R  Resistance=10000  Inductance=1e-3  SetiL0=off  InitialCurrent=0  Capacitance=1e-6  Setx0=off  InitialVoltage=0  Measurements=None
  RfA : powerlib/Elements/Series RLC Branch  DialogController=POWERSYS.PowerSysDialog  PhysicalDomain=powersysdomain  SubClassName=unknown  LeftPortType=p1  RightPortType=p1  LConnTagsString=__new0  RConnTagsString=__new0  BranchType=R  Resistance=faultR  Inductance=1e-3  SetiL0=off  InitialCurrent=0  Capacitance=1e-6  Setx0=off  InitialVoltage=0  Measurements=None
  RfB : powerlib/Elements/Series RLC Branch  DialogController=POWERSYS.PowerSysDialog  PhysicalDomain=powersysdomain  SubClassName=unknown  LeftPortType=p1  RightPortType=p1  LConnTagsString=__new0  RConnTagsString=__new0  BranchType=R  Resistance=faultR  Inductance=1e-3  SetiL0=off  InitialCurrent=0  Capacitance=1e-6  Setx0=off  InitialVoltage=0  Measurements=None
  RfC : powerlib/Elements/Series RLC Branch  DialogController=POWERSYS.PowerSysDialog  PhysicalDomain=powersysdomain  SubClassName=unknown  LeftPortType=p1  RightPortType=p1  LConnTagsString=__new0  RConnTagsString=__new0  BranchType=R  Resistance=faultR  Inductance=1e-3  SetiL0=off  InitialCurrent=0  Capacitance=1e-6  Setx0=off  InitialVoltage=0  Measurements=None
  A : PMIOPort  Tag=PMCPort  Port=1  Side=Left
  B : PMIOPort  Tag=PMCPort  Port=2  Side=Left
  C : PMIOPort  Tag=PMCPort  Port=3  Side=Left
  wires:
  &2/1 -> BreakerC/1
  &1/1 -> BreakerB/1
  &/1 -> BreakerA/1
  &3/1 -> BreakerN/1
  Tfault/1 -> &/2, &1/2, &2/2, &3/2
  faultG/1 -> &3/1
  faultC/1 -> &2/1
  faultB/1 -> &1/1
  faultA/1 -> &/1
  connections:
  RN/RConn1 -- Ground/LConn1 -- BreakerN/RConn1
  RfC/RConn1 -- RfA/RConn1 -- RfB/RConn1 -- RN/LConn1 -- BreakerN/LConn1
  BreakerA/RConn1 -- RfA/LConn1 -- RA/RConn1
  BreakerB/RConn1 -- RfB/LConn1 -- RB/RConn1
  RfC/LConn1 -- RC/RConn1 -- BreakerC/RConn1
  BreakerC/LConn1 -- C/RConn1 -- RC/LConn1
  RA/LConn1 -- BreakerA/LConn1 -- A/RConn1
  BreakerB/LConn1 -- RB/LConn1 -- B/RConn1

== system OORT/On-Line Analysis/Line 3/Fault Selector ==
  "  " : Constant  Value=faultType
  "  +" : Logic  Operator=OR  Inputs=7
  " +" : Logic  Operator=OR  Inputs=5
  + : Logic  Operator=OR  Inputs=5
  "+ " : Logic  Operator=OR  Inputs=6
  A-B-C : Fcn  Expr=(u(1)==8)
  A-B-C-G : Fcn  Expr=(u(1)==9)
  A-G : Fcn  Expr=(u(1)==1)
  B-C : Fcn  Expr=(u(1)==4)
  B-C-G : Fcn  Expr=(u(1)==5)
  B-G : Fcn  Expr=(u(1)==2)
  C-A : Fcn  Expr=(u(1)==6)
  C-A-G : Fcn  Expr=(u(1)==7)
  C-G : Fcn  Expr=(u(1)==3)
  faultA : Outport  InitialOutput=0
  faultB : Outport  Port=2  InitialOutput=0
  faultC : Outport  Port=3  InitialOutput=0
  faultG : Outport  Port=4  InitialOutput=0
  wires:
  A-B-C/1 -> +/4, "  +"/6, " +"/4
  A-B-C-G/1 -> +/5, "+ "/6, "  +"/7, " +"/5
  C-A-G/1 -> +/3, "+ "/5, "  +"/5
  C-G/1 -> "+ "/3, "  +"/1
  B-C-G/1 -> " +"/3, "+ "/4, "  +"/3
  B-C/1 -> " +"/2, "  +"/2
  B-G/1 -> "+ "/2, " +"/1
  C-A/1 -> +/2, "  +"/4
  A-G/1 -> +/1, "+ "/1
  "+ "/1 -> faultG/1
  "  +"/1 -> faultC/1
  " +"/1 -> faultB/1
  +/1 -> faultA/1
  "  "/1 -> B-C-G/1, A-B-C-G/1, A-B-C/1, C-A-G/1, C-A/1, B-C/1, B-G/1, A-G/1, C-G/1

== system OORT/On-Line Analysis/OR-1/Overcurrent Relay Scheme ==
  note: Overcurrent Relay Scheme
  Iabc : Inport
  "Analog filtering, signal  conditioning" : Subsystem
  Demux : Demux  Outputs=3
  Logic Matrix : Subsystem
  Phase A : Subsystem
  Phase B : Subsystem
  Phase C : Subsystem
  Residual : Subsystem
  Tripping Logic : Subsystem
  tm1 : Terminator
  "TRIP " : Outport  InitialOutput=0
  Logic : Outport  Port=2  InitialOutput=0
  FaultType : Outport  Port=3  InitialOutput=0
  wires:
  Iabc/1 -> "Analog filtering, signal  conditioning"/1(Iin)
  Tripping Logic/1(TRIP) -> "TRIP "/1
  Tripping Logic/2(Logic Signals) -> Logic/1
  "Analog filtering, signal  conditioning"/1(If) -> Demux/1
  Demux/1 -> Phase A/1(IA)
  "Analog filtering, signal  conditioning"/2(If0) -> Residual/1(IR)
  Demux/2 -> Phase B/1(IB)
  Demux/3 -> Phase C/1(IC)
  Phase A/1(Pickup) -> Logic Matrix/1(A)
  Phase B/1(Pickup) -> Logic Matrix/2(B)
  Phase C/1(Pickup) -> Logic Matrix/3(C)
  Residual/1(Pickup) -> Logic Matrix/4(R), Tripping Logic/2(IR)
  Logic Matrix/1(" Op") -> Tripping Logic/1(Op)
  Logic Matrix/2(Fault Type) -> FaultType/1
  "Analog filtering, signal  conditioning"/3(if) -> tm1/1

== system OORT/On-Line Analysis/OR-2/Overcurrent Relay Scheme ==
  note: Overcurrent Relay Scheme
  Iabc : Inport
  "Analog filtering, signal  conditioning" : Subsystem
  Demux : Demux  Outputs=3
  Logic Matrix : Subsystem
  Phase A : Subsystem
  Phase B : Subsystem
  Phase C : Subsystem
  Residual : Subsystem
  Tripping Logic : Subsystem
  tm1 : Terminator
  "TRIP " : Outport  InitialOutput=0
  Logic : Outport  Port=2  InitialOutput=0
  FaultType : Outport  Port=3  InitialOutput=0
  wires:
  "Analog filtering, signal  conditioning"/3(if) -> tm1/1
  Logic Matrix/2(Fault Type) -> FaultType/1
  Logic Matrix/1(" Op") -> Tripping Logic/1(Op)
  Residual/1(Pickup) -> Tripping Logic/2(IR), Logic Matrix/4(R)
  Phase C/1(Pickup) -> Logic Matrix/3(C)
  Phase B/1(Pickup) -> Logic Matrix/2(B)
  Phase A/1(Pickup) -> Logic Matrix/1(A)
  Demux/3 -> Phase C/1(IC)
  Demux/2 -> Phase B/1(IB)
  "Analog filtering, signal  conditioning"/2(If0) -> Residual/1(IR)
  Demux/1 -> Phase A/1(IA)
  "Analog filtering, signal  conditioning"/1(If) -> Demux/1
  Tripping Logic/2(Logic Signals) -> Logic/1
  Tripping Logic/1(TRIP) -> "TRIP "/1
  Iabc/1 -> "Analog filtering, signal  conditioning"/1(Iin)

== system OORT/On-Line Analysis/OR-3/Overcurrent Relay Scheme ==
  note: Overcurrent Relay Scheme
  Iabc : Inport
  "Analog filtering, signal  conditioning" : Subsystem
  Demux : Demux  Outputs=3
  Logic Matrix : Subsystem
  Phase A : Subsystem
  Phase B : Subsystem
  Phase C : Subsystem
  Residual : Subsystem
  Tripping Logic : Subsystem
  tm1 : Terminator
  "TRIP " : Outport  InitialOutput=0
  Logic : Outport  Port=2  InitialOutput=0
  FaultType : Outport  Port=3  InitialOutput=0
  wires:
  Iabc/1 -> "Analog filtering, signal  conditioning"/1(Iin)
  Tripping Logic/1(TRIP) -> "TRIP "/1
  Tripping Logic/2(Logic Signals) -> Logic/1
  "Analog filtering, signal  conditioning"/1(If) -> Demux/1
  Demux/1 -> Phase A/1(IA)
  "Analog filtering, signal  conditioning"/2(If0) -> Residual/1(IR)
  Demux/2 -> Phase B/1(IB)
  Demux/3 -> Phase C/1(IC)
  Phase A/1(Pickup) -> Logic Matrix/1(A)
  Phase B/1(Pickup) -> Logic Matrix/2(B)
  Phase C/1(Pickup) -> Logic Matrix/3(C)
  Residual/1(Pickup) -> Logic Matrix/4(R), Tripping Logic/2(IR)
  Logic Matrix/1(" Op") -> Tripping Logic/1(Op)
  Logic Matrix/2(Fault Type) -> FaultType/1
  "Analog filtering, signal  conditioning"/3(if) -> tm1/1

== system OORT/On-Line Analysis/OR-1/Overcurrent Relay Scheme/Analog filtering, signal  conditioning ==
  note: Acquisition Block- analog filtering,
      | signal conditioning, sampling.
  Iin : Inport
  CURRENTS : Subsystem
  Mux3 : Mux  Inputs=3
  Mux4 : Mux  Inputs=3
  If : Outport  InitialOutput=0
  If0 : Outport  Port=2  InitialOutput=0
  if : Outport  Port=3  InitialOutput=0
  wires:
  Iin/1 -> CURRENTS/1(Iabc)
  CURRENTS/1(IAf) -> Mux3/1
  CURRENTS/2(IBf) -> Mux3/2
  CURRENTS/3(ICf) -> Mux3/3
  CURRENTS/5(iaf) -> Mux4/1
  CURRENTS/6(ibf) -> Mux4/2
  CURRENTS/7(icf) -> Mux4/3
  Mux3/1 -> If/1
  Mux4/1 -> if/1
  CURRENTS/4(I0f) -> If0/1

== system OORT/On-Line Analysis/OR-1/Overcurrent Relay Scheme/Logic Matrix ==
  note: Overcurrent Relay - Logic Signal Matrix
  A : Inport
  B : Inport  Port=2
  C : Inport  Port=3
  R : Inport  Port=4
  Mux5 : Mux
  Op : Logic  Operator=OR  Inputs=3
  " Op" : Outport  InitialOutput=0
  Fault Type : Outport  Port=2  InitialOutput=0
  wires:
  Op/1 -> " Op"/1
  Mux5/1 -> Fault Type/1
  R/1 -> Mux5/4
  A/1 -> Mux5/1, Op/1
  B/1 -> Mux5/2, Op/2
  C/1 -> Mux5/3, Op/3

== system OORT/On-Line Analysis/OR-1/Overcurrent Relay Scheme/Phase A ==
  IA : Inport
  Integrator : Integrator
  Operation : Subsystem  mask(Zone){Ip=Iop}
      mask prompts: Ip "PhaseCurrent [A]"
  TRIP output contact : Relay  OnSwitchValue=0.9999  OffSwitchValue=-1
  delay : RelationalOperator  Operator=>  InputSameDT=on
  time delay : Constant  Value=Td+0.001
  Pickup : Outport  InitialOutput=0
  wires:
  IA/1 -> Operation/1(Iin)
  Integrator/1 -> delay/1
  time delay/1 -> delay/2
  delay/1 -> TRIP output contact/1
  Operation/1(TRIP) -> Integrator/1
  TRIP output contact/1 -> Pickup/1

== system OORT/On-Line Analysis/OR-1/Overcurrent Relay Scheme/Phase B ==
  IB : Inport
  Integrator : Integrator
  Operation : Subsystem  mask(Zone){Ip=Iop}
      mask prompts: Ip "PhaseCurrent [A]"
  TRIP output contact : Relay  OnSwitchValue=0.9999  OffSwitchValue=-1
  delay : RelationalOperator  Operator=>  InputSameDT=on
  time delay : Constant  Value=Td+0.001
  Pickup : Outport  InitialOutput=0
  wires:
  IB/1 -> Operation/1(Iin)
  Integrator/1 -> delay/1
  time delay/1 -> delay/2
  delay/1 -> TRIP output contact/1
  Operation/1(TRIP) -> Integrator/1
  TRIP output contact/1 -> Pickup/1

== system OORT/On-Line Analysis/OR-1/Overcurrent Relay Scheme/Phase C ==
  IC : Inport
  Integrator : Integrator
  Operation : Subsystem  mask(Zone){Ip=Iop}
      mask prompts: Ip "PhaseCurrent [A]"
  TRIP output contact : Relay  OnSwitchValue=0.9999  OffSwitchValue=-1
  delay : RelationalOperator  Operator=>  InputSameDT=on
  time delay : Constant  Value=Td+0.001
  Pickup : Outport  InitialOutput=0
  wires:
  IC/1 -> Operation/1(Iin)
  Integrator/1 -> delay/1
  time delay/1 -> delay/2
  delay/1 -> TRIP output contact/1
  Operation/1(TRIP) -> Integrator/1
  TRIP output contact/1 -> Pickup/1

== system OORT/On-Line Analysis/OR-1/Overcurrent Relay Scheme/Residual ==
  IR : Inport
  Integrator : Integrator
  ResCurr : Subsystem  mask(Zone){Ip=ResCurr}
      mask prompts: Ip "PhaseCurrent [A]"
  TRIP output contact : Relay  OnSwitchValue=0.9999  OffSwitchValue=-1
  delay : RelationalOperator  Operator=>  InputSameDT=on
  time delay : Constant  Value=Td+0.001
  Pickup : Outport  InitialOutput=0
  wires:
  IR/1 -> ResCurr/1(Iin)
  Integrator/1 -> delay/1
  time delay/1 -> delay/2
  delay/1 -> TRIP output contact/1
  ResCurr/1(TRIP) -> Integrator/1
  TRIP output contact/1 -> Pickup/1

== system OORT/On-Line Analysis/OR-1/Overcurrent Relay Scheme/Tripping Logic ==
  note: Overcurrent Relay - Tripping Logic
  Op : Inport
  IR : Inport  Port=2
  Add : Sum
  Constant : Constant  Value=2
  Mux : Mux  Inputs=2
  TRIP : Outport  InitialOutput=0
  Logic Signals : Outport  Port=2  InitialOutput=0
  wires:
  Mux/1 -> Logic Signals/1
  Op/1 -> Add/1, TRIP/1
  Add/1 -> Mux/2
  Constant/1 -> Add/2
  IR/1 -> Mux/1

== system OORT/On-Line Analysis/OR-2/Overcurrent Relay Scheme/Analog filtering, signal  conditioning ==
  note: Acquisition Block- analog filtering,
      | signal conditioning, sampling.
  Iin : Inport
  CURRENTS : Subsystem
  Mux3 : Mux  Inputs=3
  Mux4 : Mux  Inputs=3
  If : Outport  InitialOutput=0
  If0 : Outport  Port=2  InitialOutput=0
  if : Outport  Port=3  InitialOutput=0
  wires:
  CURRENTS/4(I0f) -> If0/1
  Mux4/1 -> if/1
  Mux3/1 -> If/1
  CURRENTS/7(icf) -> Mux4/3
  CURRENTS/6(ibf) -> Mux4/2
  CURRENTS/5(iaf) -> Mux4/1
  CURRENTS/3(ICf) -> Mux3/3
  CURRENTS/2(IBf) -> Mux3/2
  CURRENTS/1(IAf) -> Mux3/1
  Iin/1 -> CURRENTS/1(Iabc)

== system OORT/On-Line Analysis/OR-2/Overcurrent Relay Scheme/Logic Matrix ==
  note: Overcurrent Relay - Logic Signal Matrix
  A : Inport
  B : Inport  Port=2
  C : Inport  Port=3
  R : Inport  Port=4
  Mux5 : Mux
  Op : Logic  Operator=OR  Inputs=3
  " Op" : Outport  InitialOutput=0
  Fault Type : Outport  Port=2  InitialOutput=0
  wires:
  C/1 -> Op/3, Mux5/3
  B/1 -> Op/2, Mux5/2
  A/1 -> Op/1, Mux5/1
  R/1 -> Mux5/4
  Mux5/1 -> Fault Type/1
  Op/1 -> " Op"/1

== system OORT/On-Line Analysis/OR-2/Overcurrent Relay Scheme/Phase A ==
  IA : Inport
  Integrator : Integrator
  Operation : Subsystem  mask(Zone){Ip=Iop}
      mask prompts: Ip "PhaseCurrent [A]"
  TRIP output contact : Relay  OnSwitchValue=0.9999  OffSwitchValue=-1
  delay : RelationalOperator  Operator=>  InputSameDT=on
  time delay : Constant  Value=Td+0.001
  Pickup : Outport  InitialOutput=0
  wires:
  TRIP output contact/1 -> Pickup/1
  Operation/1(TRIP) -> Integrator/1
  delay/1 -> TRIP output contact/1
  time delay/1 -> delay/2
  Integrator/1 -> delay/1
  IA/1 -> Operation/1(Iin)

== system OORT/On-Line Analysis/OR-2/Overcurrent Relay Scheme/Phase B ==
  IB : Inport
  Integrator : Integrator
  Operation : Subsystem  mask(Zone){Ip=Iop}
      mask prompts: Ip "PhaseCurrent [A]"
  TRIP output contact : Relay  OnSwitchValue=0.9999  OffSwitchValue=-1
  delay : RelationalOperator  Operator=>  InputSameDT=on
  time delay : Constant  Value=Td+0.001
  Pickup : Outport  InitialOutput=0
  wires:
  TRIP output contact/1 -> Pickup/1
  Operation/1(TRIP) -> Integrator/1
  delay/1 -> TRIP output contact/1
  time delay/1 -> delay/2
  Integrator/1 -> delay/1
  IB/1 -> Operation/1(Iin)

== system OORT/On-Line Analysis/OR-2/Overcurrent Relay Scheme/Phase C ==
  IC : Inport
  Integrator : Integrator
  Operation : Subsystem  mask(Zone){Ip=Iop}
      mask prompts: Ip "PhaseCurrent [A]"
  TRIP output contact : Relay  OnSwitchValue=0.9999  OffSwitchValue=-1
  delay : RelationalOperator  Operator=>  InputSameDT=on
  time delay : Constant  Value=Td+0.001
  Pickup : Outport  InitialOutput=0
  wires:
  TRIP output contact/1 -> Pickup/1
  Operation/1(TRIP) -> Integrator/1
  delay/1 -> TRIP output contact/1
  time delay/1 -> delay/2
  Integrator/1 -> delay/1
  IC/1 -> Operation/1(Iin)

== system OORT/On-Line Analysis/OR-2/Overcurrent Relay Scheme/Residual ==
  IR : Inport
  Integrator : Integrator
  ResCurr : Subsystem  mask(Zone){Ip=ResCurr}
      mask prompts: Ip "PhaseCurrent [A]"
  TRIP output contact : Relay  OnSwitchValue=0.9999  OffSwitchValue=-1
  delay : RelationalOperator  Operator=>  InputSameDT=on
  time delay : Constant  Value=Td+0.001
  Pickup : Outport  InitialOutput=0
  wires:
  TRIP output contact/1 -> Pickup/1
  ResCurr/1(TRIP) -> Integrator/1
  delay/1 -> TRIP output contact/1
  time delay/1 -> delay/2
  Integrator/1 -> delay/1
  IR/1 -> ResCurr/1(Iin)

== system OORT/On-Line Analysis/OR-2/Overcurrent Relay Scheme/Tripping Logic ==
  note: Overcurrent Relay - Tripping Logic
  Op : Inport
  IR : Inport  Port=2
  Add : Sum
  Constant : Constant  Value=2
  Mux : Mux  Inputs=2
  TRIP : Outport  InitialOutput=0
  Logic Signals : Outport  Port=2  InitialOutput=0
  wires:
  IR/1 -> Mux/1
  Constant/1 -> Add/2
  Add/1 -> Mux/2
  Op/1 -> TRIP/1, Add/1
  Mux/1 -> Logic Signals/1

== system OORT/On-Line Analysis/OR-3/Overcurrent Relay Scheme/Analog filtering, signal  conditioning ==
  note: Acquisition Block- analog filtering,
      | signal conditioning, sampling.
  Iin : Inport
  CURRENTS : Subsystem
  Mux3 : Mux  Inputs=3
  Mux4 : Mux  Inputs=3
  If : Outport  InitialOutput=0
  If0 : Outport  Port=2  InitialOutput=0
  if : Outport  Port=3  InitialOutput=0
  wires:
  Iin/1 -> CURRENTS/1(Iabc)
  CURRENTS/1(IAf) -> Mux3/1
  CURRENTS/2(IBf) -> Mux3/2
  CURRENTS/3(ICf) -> Mux3/3
  CURRENTS/5(iaf) -> Mux4/1
  CURRENTS/6(ibf) -> Mux4/2
  CURRENTS/7(icf) -> Mux4/3
  Mux3/1 -> If/1
  Mux4/1 -> if/1
  CURRENTS/4(I0f) -> If0/1

== system OORT/On-Line Analysis/OR-3/Overcurrent Relay Scheme/Logic Matrix ==
  note: Overcurrent Relay - Logic Signal Matrix
  A : Inport
  B : Inport  Port=2
  C : Inport  Port=3
  R : Inport  Port=4
  Mux5 : Mux
  Op : Logic  Operator=OR  Inputs=3
  " Op" : Outport  InitialOutput=0
  Fault Type : Outport  Port=2  InitialOutput=0
  wires:
  Op/1 -> " Op"/1
  Mux5/1 -> Fault Type/1
  R/1 -> Mux5/4
  A/1 -> Mux5/1, Op/1
  B/1 -> Mux5/2, Op/2
  C/1 -> Mux5/3, Op/3

== system OORT/On-Line Analysis/OR-3/Overcurrent Relay Scheme/Phase A ==
  IA : Inport
  Integrator : Integrator
  Operation : Subsystem  mask(Zone){Ip=Iop}
      mask prompts: Ip "PhaseCurrent [A]"
  TRIP output contact : Relay  OnSwitchValue=0.9999  OffSwitchValue=-1
  delay : RelationalOperator  Operator=>  InputSameDT=on
  time delay : Constant  Value=Td+0.001
  Pickup : Outport  InitialOutput=0
  wires:
  IA/1 -> Operation/1(Iin)
  Integrator/1 -> delay/1
  time delay/1 -> delay/2
  delay/1 -> TRIP output contact/1
  Operation/1(TRIP) -> Integrator/1
  TRIP output contact/1 -> Pickup/1

== system OORT/On-Line Analysis/OR-3/Overcurrent Relay Scheme/Phase B ==
  IB : Inport
  Integrator : Integrator
  Operation : Subsystem  mask(Zone){Ip=Iop}
      mask prompts: Ip "PhaseCurrent [A]"
  TRIP output contact : Relay  OnSwitchValue=0.9999  OffSwitchValue=-1
  delay : RelationalOperator  Operator=>  InputSameDT=on
  time delay : Constant  Value=Td+0.001
  Pickup : Outport  InitialOutput=0
  wires:
  IB/1 -> Operation/1(Iin)
  Integrator/1 -> delay/1
  time delay/1 -> delay/2
  delay/1 -> TRIP output contact/1
  Operation/1(TRIP) -> Integrator/1
  TRIP output contact/1 -> Pickup/1

== system OORT/On-Line Analysis/OR-3/Overcurrent Relay Scheme/Phase C ==
  IC : Inport
  Integrator : Integrator
  Operation : Subsystem  mask(Zone){Ip=Iop}
      mask prompts: Ip "PhaseCurrent [A]"
  TRIP output contact : Relay  OnSwitchValue=0.9999  OffSwitchValue=-1
  delay : RelationalOperator  Operator=>  InputSameDT=on
  time delay : Constant  Value=Td+0.001
  Pickup : Outport  InitialOutput=0
  wires:
  IC/1 -> Operation/1(Iin)
  Integrator/1 -> delay/1
  time delay/1 -> delay/2
  delay/1 -> TRIP output contact/1
  Operation/1(TRIP) -> Integrator/1
  TRIP output contact/1 -> Pickup/1

== system OORT/On-Line Analysis/OR-3/Overcurrent Relay Scheme/Residual ==
  IR : Inport
  Integrator : Integrator
  ResCurr : Subsystem  mask(Zone){Ip=ResCurr}
      mask prompts: Ip "PhaseCurrent [A]"
  TRIP output contact : Relay  OnSwitchValue=0.9999  OffSwitchValue=-1
  delay : RelationalOperator  Operator=>  InputSameDT=on
  time delay : Constant  Value=Td+0.001
  Pickup : Outport  InitialOutput=0
  wires:
  IR/1 -> ResCurr/1(Iin)
  Integrator/1 -> delay/1
  time delay/1 -> delay/2
  delay/1 -> TRIP output contact/1
  ResCurr/1(TRIP) -> Integrator/1
  TRIP output contact/1 -> Pickup/1

== system OORT/On-Line Analysis/OR-3/Overcurrent Relay Scheme/Tripping Logic ==
  note: Overcurrent Relay - Tripping Logic
  Op : Inport
  IR : Inport  Port=2
  Add : Sum
  Constant : Constant  Value=2
  Mux : Mux  Inputs=2
  TRIP : Outport  InitialOutput=0
  Logic Signals : Outport  Port=2  InitialOutput=0
  wires:
  Mux/1 -> Logic Signals/1
  Op/1 -> Add/1, TRIP/1
  Add/1 -> Mux/2
  Constant/1 -> Add/2
  IR/1 -> Mux/1
